simulink model "PI_regulator"  (R2023a)
settings: Solver=VariableStepAuto  StartTime=0.0  StopTime=100  RelTol=1e-3
libraries: simulink x1
settings Model: Creator=levsi  LastModifiedBy=levsi
settings SolverCC: ZeroCrossAlgorithm=Adaptive
settings DebuggingCC: IgnoredZcDiagnostic=none

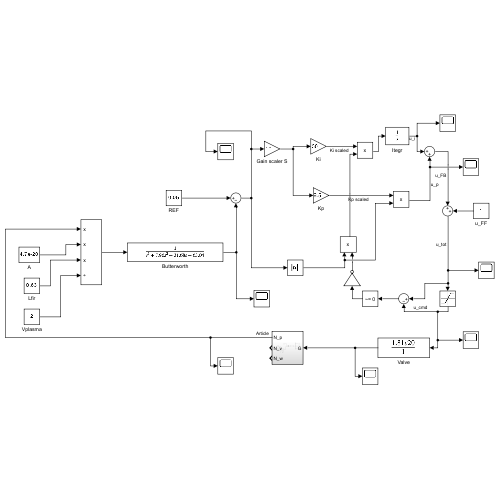
[thumbnail: Simulink's stored preview of the top-level diagram]
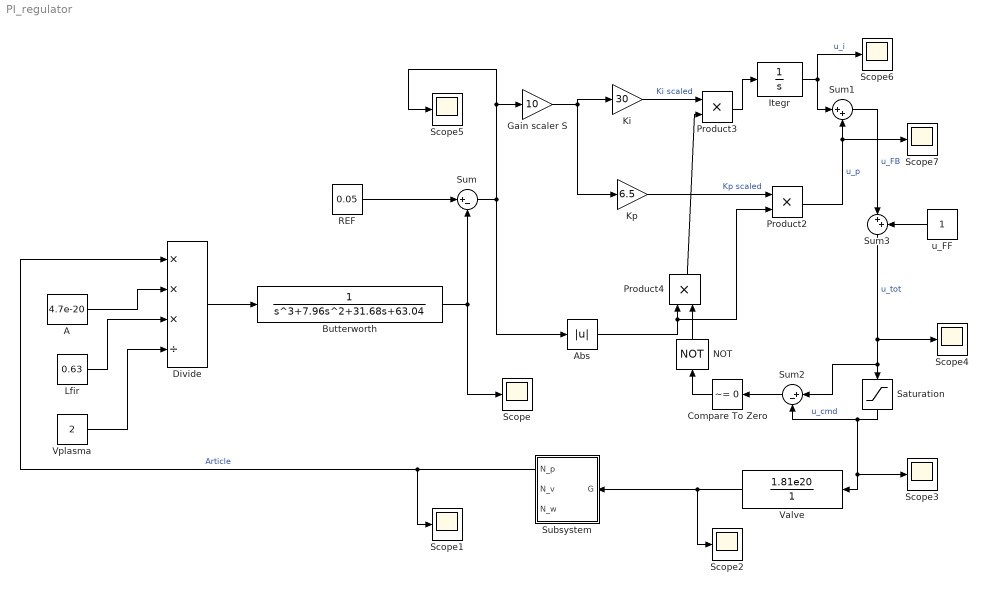
== system PI_regulator ==
  A : Constant  Value=4.7e-20
  Abs : Abs  SaturateOnIntegerOverflow=off
  Butterworth : TransferFcn  Denominator=[1 7.96 31.68 63.04]
  Compare To Zero : simulink/Logic and Bit Operations/Compare To Zero  relop=~=  OutDataTypeStr=boolean
  Divide : Product  Inputs=***/
  Gain scaler S : Gain  Gain=10
  Itegr : TransferFcn  Denominator=[1 0]
  Ki : Gain  Gain=30
  Kp : Gain  Gain=6.5
  Lfir : Constant  Value=0.63
  NOT : Logic  Operator=NOT  IconShape=distinctive  AllPortsSameDT=off  OutDataTypeStr=boolean
  Product2 : Product
  Product3 : Product
  Product4 : Product
  REF : Constant  Value=0.05
  Saturation : Saturate  UpperLimit=10  LowerLimit=0
  Scope{,1..7} (8 alike) : Scope
  Subsystem : Subsystem
  Sum : Sum  Inputs=|+-
  Sum1 : Sum  Inputs=|++
  Sum2 : Sum  Inputs=|+-
  Sum3 : Sum  Inputs=|++
  Valve : TransferFcn  Numerator=[1.81e20]  Denominator=[1]
  Vplasma : Constant  Value=2
  u_FF : Constant
  wires:
  Vplasma/1 -> Divide/4
  Lfir/1 -> Divide/3
  A/1 -> Divide/2
  Divide/1 -> Butterworth/1
  Butterworth/1 -> Scope/1, Sum/2
  Sum/1 -> Abs/1, Scope5/1, Gain scaler S/1
  Gain scaler S/1 -> Kp/1, Ki/1
  Kp/1 -> Product2/1  "Kp scaled"
  Product2/1 -> Sum1/2, Scope7/1  "u_p"
  Ki/1 -> Product3/1  "Ki scaled"
  Product4/1 -> Product3/2
  Itegr/1 -> Scope6/1, Sum1/1  "u_i"
  Product3/1 -> Itegr/1
  NOT/1 -> Product4/2
  Compare To Zero/1 -> NOT/1
  Sum2/1 -> Compare To Zero/1
  Sum1/1 -> Sum3/1  "u_FB"
  u_FF/1 -> Sum3/2
  Sum3/1 -> Scope4/1, Sum2/1, Saturation/1  "u_tot"
  Saturation/1 -> Scope3/1, Valve/1, Sum2/2  "u_cmd"
  Valve/1 -> Scope2/1, Subsystem/1(G)
  Subsystem/1(N_p) -> Scope1/1, Divide/1  "Article"
  REF/1 -> Sum/1
  Abs/1 -> Product2/2, Product4/1

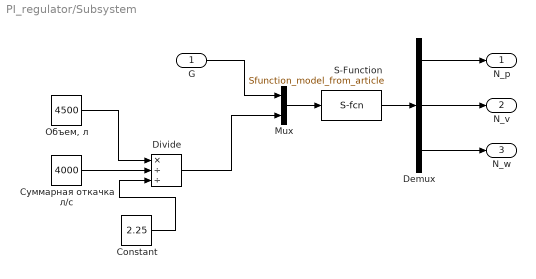
== system PI_regulator/Subsystem ==
  G : Inport
  Constant : Constant  Value=2.25
  Demux : Demux  Outputs=3
  Divide : Product  Inputs=*//
  Mux : Mux  Inputs=2
  S-Function : S-Function  FunctionName=Sfunction_model_from_article  Parameters=0.018, 0.01, 0.283, 0.041, 0, 0, 2.5e+18  SFunctionDeploymentMode=off  EnableBusSupport=off
  "Объем, л" : Constant  Value=4500
  Суммарная откачка л/с : Constant  Value=4000
  N_p : Outport
  N_v : Outport  Port=2
  N_w : Outport  Port=3
  wires:
  Demux/1 -> N_p/1
  S-Function/1 -> Demux/1
  Demux/2 -> N_v/1
  Demux/3 -> N_w/1
  Mux/1 -> S-Function/1
  G/1 -> Mux/1
  Divide/1 -> Mux/2
  Constant/1 -> Divide/3
  Суммарная откачка л/с/1 -> Divide/2
  "Объем, л"/1 -> Divide/1
